simulink model "exothermalCSTR_LinearSS"  (R2017a)
settings: Solver=VariableStepAuto  StartTime=0.0  StopTime=500.0  RelTol=1e-3
values from neighbouring files (symbols this model uses):
  A = A_e(U_ss(idx,:), X_ss(idx,idx,:))    [exo_cstr_main.m]
  B = B_e(U_ss(idx,:), X_ss(idx,idx,:))    [exo_cstr_main.m]
  cA_ss = X_ss(idx,idx,1)    [exo_cstr_main.m]
  cB_ss = X_ss(idx,idx,2)    [exo_cstr_main.m]
  T_ss = X_ss(idx,idx,3)    [exo_cstr_main.m]
  Tc_ss = X_ss(idx,idx,4)    [exo_cstr_main.m]
  U1_ss = U_ss(idx,1)    [exo_cstr_main.m]
  U2_ss = U_ss(idx,2)    [exo_cstr_main.m]
  y0 = [cA_ss cB_ss T_ss Tc_ss]    [exo_cstr_main.m]
settings Model: Creator=minhotmog  LastModifiedBy=minhotmog

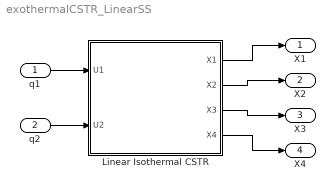
== system exothermalCSTR_LinearSS ==
  q1 : Inport
  q2 : Inport  Port=2
  Linear Isothermal CSTR : Subsystem
  X1 : Outport
  X2 : Outport  Port=2
  X3 : Outport  Port=3
  X4 : Outport  Port=4
  wires:
  Linear Isothermal CSTR/1(X1) -> X1/1
  Linear Isothermal CSTR/2(X2) -> X2/1
  Linear Isothermal CSTR/3(X3) -> X3/1
  q1/1 -> Linear Isothermal CSTR/1(U1)
  Linear Isothermal CSTR/4(X4) -> X4/1
  q2/1 -> Linear Isothermal CSTR/2(U2)

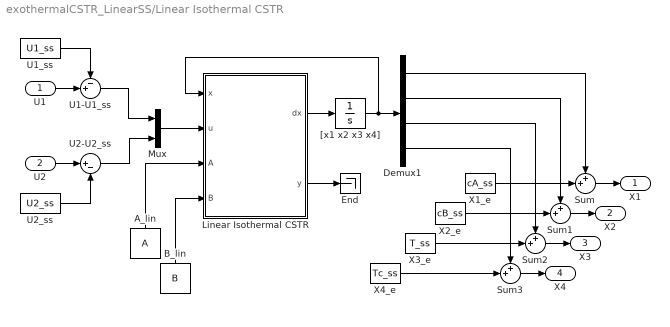
== system exothermalCSTR_LinearSS/Linear Isothermal CSTR ==
  U1 : Inport
  U2 : Inport  Port=2
  A_lin : Constant  Value=A
  B_lin : Constant  Value=B
  Demux1 : Demux
  End : Terminator
  Linear Isothermal CSTR : MATLAB Function  TreatAsAtomicUnit=on
  Mux : Mux  Inputs=2
  Sum{,1..3} (4 alike) : Sum  Inputs=++|
  U1-U1_ss : Sum  Inputs=-+|
  U1_ss : Constant  Value=U1_ss
  U2-U2_ss : Sum  Inputs=|+-
  U2_ss : Constant  Value=U2_ss
  X1_e : Constant  Value=cA_ss
  X2_e : Constant  Value=cB_ss
  X3_e : Constant  Value=T_ss
  X4_e : Constant  Value=Tc_ss
  "[x1 x2 x3 x4]" : Integrator  InitialCondition=[y0(1)-cA_ss y0(2)-cB_ss y0(3)-T_ss y0(4)-Tc_ss]  UpperSaturationLimit=[0.6 0.6 0.6]  LowerSaturationLimit=[0 0 0]
  X1 : Outport
  X2 : Outport  Port=2
  X3 : Outport  Port=3
  X4 : Outport  Port=4
  wires:
  U1-U1_ss/1 -> Mux/1
  "[x1 x2 x3 x4]"/1 -> Linear Isothermal CSTR/1(x), Demux1/1
  Linear Isothermal CSTR/1(dx) -> "[x1 x2 x3 x4]"/1
  U1/1 -> U1-U1_ss/2
  U1_ss/1 -> U1-U1_ss/1
  X1_e/1 -> Sum/2
  X2_e/1 -> Sum1/2
  X3_e/1 -> Sum2/2
  A_lin/1 -> Linear Isothermal CSTR/3(A)
  Linear Isothermal CSTR/2(y) -> End/1
  X4_e/1 -> Sum3/2
  B_lin/1 -> Linear Isothermal CSTR/4(B)
  Sum3/1 -> X4/1
  Sum2/1 -> X3/1
  Sum1/1 -> X2/1
  Sum/1 -> X1/1
  Demux1/4 -> Sum3/1
  Demux1/3 -> Sum2/1
  Demux1/2 -> Sum1/1
  Demux1/1 -> Sum/1
  Mux/1 -> Linear Isothermal CSTR/2(u)
  U2/1 -> U2-U2_ss/1
  U2_ss/1 -> U2-U2_ss/2
  U2-U2_ss/1 -> Mux/2

== matlab function exothermalCSTR_LinearSS/Linear Isothermal CSTR/Linear Isothermal CSTR ==
  data: x input; dx output; u input; y output; A input; B input
function [dx, y] = Linear_SS(x, u, A, B)
    dx = zeros(4 ,1) ;
    y = zeros(4 ,1) ;

    C = eye(4);
    
    dx = A * x + B * u;
    y  = C * x;
